simulink model "control"  (R2019a)
settings: Solver=VariableStepAuto  StartTime=0.0  StopTime=40  RelTol=1e-3
InitFcn:
  | ur5_trajectory2
settings Model: Creator=Valdir Jr  LastModifiedBy=Valdir Jr

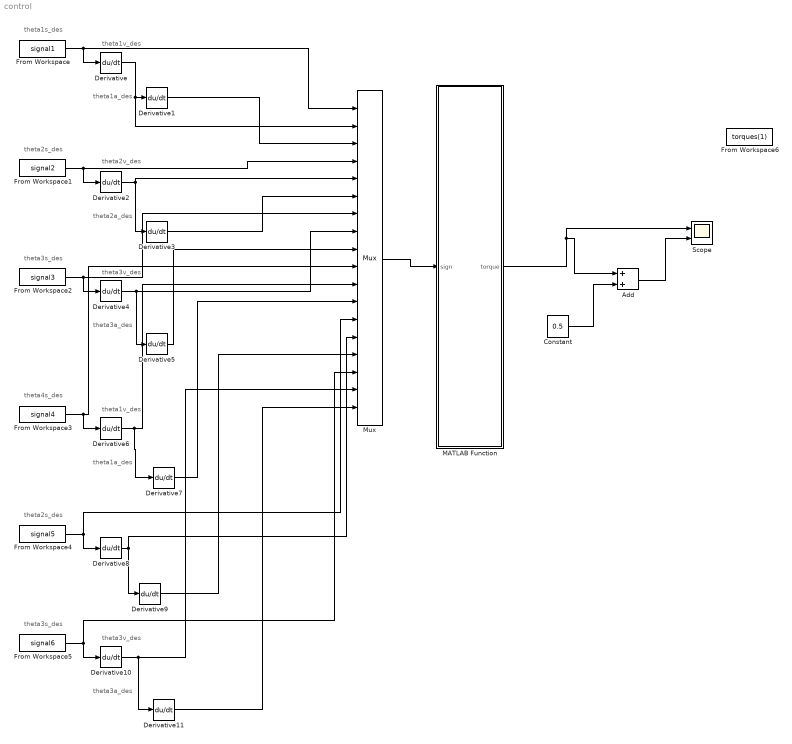
== system control ==
  note: theta1a_des
  note: theta1v_des
  note: theta1s_des
  note: theta2s_des
  note: theta2a_des
  note: theta2v_des
  note: theta3s_des
  note: theta3a_des
  note: theta3v_des
  note: theta4s_des
  note: theta1a_des
  note: theta2s_des
  note: theta1v_des
  note: theta3a_des
  note: theta3v_des
  note: theta3s_des
  Add : Sum
  Constant : Constant  Value=0.5
  Derivative{,1..11} (12 alike) : Derivative
  From Workspace : FromWorkspace  VariableName=signal1  SampleTime=0
  From Workspace1 : FromWorkspace  VariableName=signal2  SampleTime=0
  From Workspace2 : FromWorkspace  VariableName=signal3  SampleTime=0
  From Workspace3 : FromWorkspace  VariableName=signal4  SampleTime=0
  From Workspace4 : FromWorkspace  VariableName=signal5  SampleTime=0
  From Workspace5 : FromWorkspace  VariableName=signal6  SampleTime=0
  From Workspace6 : FromWorkspace  VariableName=torques(1)  SampleTime=0
  MATLAB Function : MATLAB Function  TreatAsAtomicUnit=on
  Mux : Mux  Inputs=18
  Scope : Scope  NumInputPorts=2
  wires:
  From Workspace/1 -> Mux/1, Derivative/1
  From Workspace1/1 -> Mux/4, Derivative2/1
  From Workspace2/1 -> Mux/7, Derivative4/1
  From Workspace4/1 -> Mux/13, Derivative8/1
  From Workspace5/1 -> Mux/16, Derivative10/1
  From Workspace3/1 -> Mux/10, Derivative6/1
  Derivative2/1 -> Mux/5, Derivative3/1
  Derivative4/1 -> Mux/8, Derivative5/1
  Derivative/1 -> Mux/2, Derivative1/1
  Constant/1 -> Add/2
  MATLAB Function/1(torque) -> Scope/1, Add/1
  Add/1 -> Scope/2
  Derivative6/1 -> Mux/11, Derivative7/1
  Derivative10/1 -> Mux/17, Derivative11/1
  Derivative8/1 -> Mux/14, Derivative9/1
  Derivative11/1 -> Mux/18
  Derivative9/1 -> Mux/15
  Derivative5/1 -> Mux/9
  Derivative1/1 -> Mux/3
  Derivative3/1 -> Mux/6
  Derivative7/1 -> Mux/12
  Mux/1 -> MATLAB Function/1(sign)

== matlab function control/MATLAB Function ==
  data: sign input; torque output
function torque = fcn(sign)
theta1 = sign(1);
theta1_v = sign(2);
theta1_a = sign(3);

theta2 = sign(4);
theta2_v = sign(5);
theta2_a = sign(6);

theta3 = sign(7);
theta3_v = sign(8);
theta3_a = sign(9);

theta4 = sign(10);
theta4_v = sign(11);
theta4_a = sign(12);

theta5 = sign(13);
theta5_v = sign(14);
theta5_a = sign(15);

theta6 = sign(16);
theta6_v = sign(17);
theta6_a = sign(18);
torque= (13230568142103*theta1_a)/8000000000000 + (30420299*theta2_a)/80000000 + (1923182992103*theta3_a)/8000000000000 + (16027676523*theta4_a)/800000000000 + (269901439*theta5_a)/320000000000 - (3038343*theta2_a*sin(theta2 + theta3 + theta5))/1000000000 - (1054119*theta1_a*sin(theta3 + theta4 + theta5))/320000000 - (1054119*theta3_a*sin(theta3 + theta4 + theta5))/640000000 + (38328171*theta1_a*cos(2*theta2))/32000000 + (26299*theta2_a*cos(2*theta2))/128000 + (3166231*theta1_a*cos(2*theta5))/6400000000 + (2046231*theta3_a*cos(2*theta5))/6400000000 - (1974573679*theta1_a*cos(2*theta2 + 2*theta3 + 2*theta4))/320000000000 - (1918573679*theta3_a*cos(2*theta2 + 2*theta3 + 2*theta4))/320000000000 - (175098379*theta4_a*cos(2*theta2 + 2*theta3 + 2*theta4))/32000000000 - (269901439*theta5_a*cos(2*theta2 + 2*theta3 + 2*theta4))/320000000000 + (1054119*theta1_a*sin(2*theta2 + theta3 + theta4 - theta5))/320000000 - (3038343*theta1_a*sin(2*theta2 + 2*theta3 + theta4 + theta5))/1000000000 + (1054119*theta3_a*sin(2*theta2 + theta3 + theta4 - theta5))/640000000 - (3038343*theta3_a*sin(2*theta2 + 2*theta3 + theta4 + theta5))/1000000000 + (124639359*theta1_a*cos(2*theta2 + 2*theta3))/312500000 + (218491*theta2_a*cos(2*theta2 + 2*theta3))/1250000 + (63047859*theta3_a*cos(2*theta2 + 2*theta3))/312500000 + (90646567*theta1_a*sin(2*theta2 + theta3 + theta4))/1600000000 - (3038343*theta2_a*sin(theta2 + theta3 - theta5))/1000000000 + (1054119*theta1_a*sin(theta3 + theta4 - theta5))/320000000 + (90646567*theta3_a*sin(2*theta2 + theta3 + theta4))/3200000000 + (7854017*theta4_a*sin(2*theta2 + theta3 + theta4))/320000000 + (1054119*theta3_a*sin(theta3 + theta4 - theta5))/640000000 + (12106397*theta5_a*sin(2*theta2 + theta3 + theta4))/3200000000 - (18044037*theta2_a*cos(theta2 + theta3 + theta4 + theta5))/160000000000 - (18044037*theta4_a*cos(theta2 + theta3 + theta4 + theta5))/160000000000 - (63773651*theta6_a*cos(theta2 + theta3 + theta4 + theta5))/80000000000 + (23500653*theta1_a*cos(2*theta2 + 2*theta3 + 2*theta4 + theta5))/32000000000 + (23500653*theta3_a*cos(2*theta2 + 2*theta3 + 2*theta4 + theta5))/32000000000 + (23500653*theta5_a*cos(2*theta2 + 2*theta3 + 2*theta4 + theta5))/64000000000 - (1406353263*theta2_a*sin(theta2 + theta3))/12500000000 + (90646567*theta1_a*sin(theta3 + theta4))/1600000000 - (1054119*theta2_a*sin(theta2 + theta5))/320000000 - (3038343*theta1_a*sin(theta4 + theta5))/1000000000 + (90646567*theta3_a*sin(theta3 + theta4))/3200000000 + (7854017*theta4_a*sin(theta3 + theta4))/320000000 - (3038343*theta3_a*sin(theta4 + theta5))/1000000000 + (12106397*theta5_a*sin(theta3 + theta4))/3200000000 + (3038343*theta1_a*sin(2*theta2 + 2*theta3 + theta4 - theta5))/1000000000 + (3038343*theta3_a*sin(2*theta2 + 2*theta3 + theta4 - theta5))/1000000000 + (40824497*theta1_a*cos(theta3))/50000000 + (75803*theta2_a*cos(theta3))/200000 + (67773651*theta1_a*cos(theta5))/20000000000 + (21873747*theta3_a*cos(theta3))/100000000 + (67773651*theta3_a*cos(theta5))/20000000000 - (487918479*theta2_a*sin(theta2))/4000000000 + (261275399*theta1_a*sin(theta4))/5000000000 + (261275399*theta3_a*sin(theta4))/5000000000 + (22638049*theta4_a*sin(theta4))/1000000000 + (34894909*theta5_a*sin(theta4))/10000000000 + (261275399*theta1_a*sin(2*theta2 + 2*theta3 + theta4))/5000000000 + (261275399*theta3_a*sin(2*theta2 + 2*theta3 + theta4))/5000000000 + (22638049*theta4_a*sin(2*theta2 + 2*theta3 + theta4))/1000000000 + (34894909*theta5_a*sin(2*theta2 + 2*theta3 + theta4))/10000000000 + (253050567*theta2_a*cos(theta2 + theta3 + theta4 - theta5))/160000000000 + (3166231*theta2_a*cos(theta2 + theta3 + theta4 - 2*theta5))/6400000000 - (3166231*theta2_a*cos(theta2 + theta3 + theta4 + 2*theta5))/6400000000 + (7*theta3_a*cos(theta2 + theta3 + theta4 - 2*theta5))/40000 - (7*theta3_a*cos(theta2 + theta3 + theta4 + 2*theta5))/40000 + (253050567*theta4_a*cos(theta2 + theta3 + theta4 - theta5))/160000000000 + (3166231*theta4_a*cos(theta2 + theta3 + theta4 - 2*theta5))/6400000000 - (3166231*theta4_a*cos(theta2 + theta3 + theta4 + 2*theta5))/6400000000 + (63773651*theta6_a*cos(theta2 + theta3 + theta4 - theta5))/80000000000 + (2046231*theta6_a*cos(theta2 + theta3 + theta4 - 2*theta5))/6400000000 - (2046231*theta6_a*cos(theta2 + theta3 + theta4 + 2*theta5))/6400000000 - (1054119*theta1_a*sin(2*theta2 + theta3 + theta4 + theta5))/320000000 - (1054119*theta3_a*sin(2*theta2 + theta3 + theta4 + theta5))/640000000 + (40824497*theta1_a*cos(2*theta2 + theta3))/50000000 + (75803*theta2_a*cos(2*theta2 + theta3))/200000 + (21873747*theta3_a*cos(2*theta2 + theta3))/100000000 - (23500653*theta1_a*cos(2*theta2 + 2*theta3 + 2*theta4 - theta5))/32000000000 - (3166231*theta1_a*cos(2*theta2 + 2*theta3 + 2*theta4 - 2*theta5))/12800000000 - (3166231*theta1_a*cos(2*theta2 + 2*theta3 + 2*theta4 + 2*theta5))/12800000000 - (23500653*theta3_a*cos(2*theta2 + 2*theta3 + 2*theta4 - theta5))/32000000000 - (2046231*theta3_a*cos(2*theta2 + 2*theta3 + 2*theta4 - 2*theta5))/12800000000 - (2046231*theta3_a*cos(2*theta2 + 2*theta3 + 2*theta4 + 2*theta5))/12800000000 - (23500653*theta5_a*cos(2*theta2 + 2*theta3 + 2*theta4 - theta5))/64000000000 - (1054119*theta2_a*sin(theta2 - theta5))/320000000 + (3038343*theta1_a*sin(theta4 - theta5))/1000000000 + (3038343*theta3_a*sin(theta4 - theta5))/1000000000 + (5828041043*theta2_a*cos(theta2 + theta3 + theta4))/400000000000 + (778370113*theta4_a*cos(theta2 + theta3 + theta4))/400000000000 + (436967093*theta5_a*cos(theta2 + theta3 + theta4))/40000000000
